simulink model "evse_twin_shit"  (R2023b)
settings: Solver=VariableStepAuto  StartTime=0.0  StopTime=5  RelTol=1e-3
libraries: fl_lib x14, nesl_utility x7
settings Model: Creator=dawid  LastModifiedBy=dawid
settings OptimizationCC: BooleanDataType=off

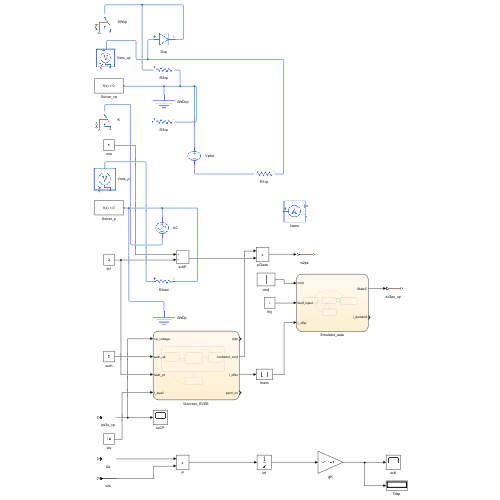
[thumbnail: Simulink's stored preview of the top-level diagram]
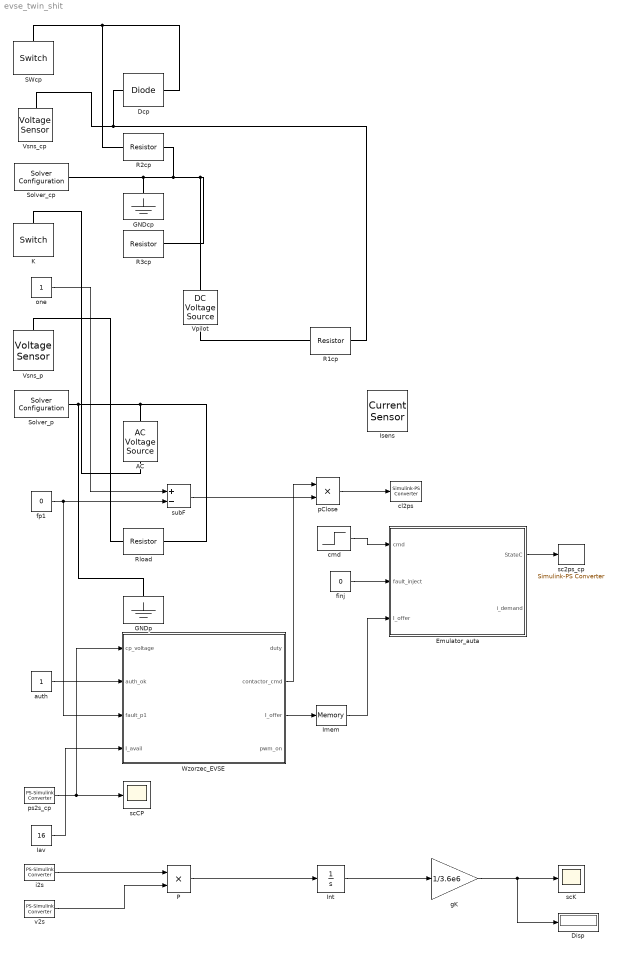
== system evse_twin_shit ==
  AC : fl_lib/Electrical/Electrical Sources/AC Voltage Source  amp=1 V  shift=0 deg  frequency=50 Hz  omega=0 rad/s
  Dcp : fl_lib/Electrical/Electrical Elements/Diode  Vf=0.6 V  Ron=0.3 Ohm  Goff=1e-8 1/Ohm  i_specify=off  i_priority=None  i=0 A  i_nominal_specify=off  i_nominal_unit=A  i_nominal_value=1  v_specify=off  v_priority=None  v=0 V  v_nominal_specify=off  v_nominal_unit=V  v_nominal_value=1
  Disp : Display
  Emulator_auta : Stateflow chart  TreatAsAtomicUnit=on
  GNDcp : fl_lib/Electrical/Electrical Elements/Electrical Reference
  GNDp : fl_lib/Electrical/Electrical Elements/Electrical Reference
  Iav : Constant  Value=16
  Imem : Memory
  Int : Integrator
  Isens : fl_lib/Electrical/Electrical Sensors/Current Sensor
  K : fl_lib/Electrical/Electrical Elements/Switch  R_closed=0.01 Ohm  G_open=1e-8 1/Ohm  Threshold=0.5  i_specify=off  i_priority=None  i=0 A  i_nominal_specify=off  i_nominal_unit=A  i_nominal_value=1  v_specify=off  v_priority=None  v=0 V  v_nominal_specify=off  v_nominal_unit=V  v_nominal_value=1
  P : Product
  R1cp : fl_lib/Electrical/Electrical Elements/Resistor  R=1000 Ohm  i_specify=off  i_priority=None  i=0 A  i_nominal_specify=off  i_nominal_unit=A  i_nominal_value=1  v_specify=off  v_priority=None  v=0 V  v_nominal_specify=off  v_nominal_unit=V  v_nominal_value=1
  R2cp : fl_lib/Electrical/Electrical Elements/Resistor  R=2740 Ohm  i_specify=off  i_priority=None  i=0 A  i_nominal_specify=off  i_nominal_unit=A  i_nominal_value=1  v_specify=off  v_priority=None  v=0 V  v_nominal_specify=off  v_nominal_unit=V  v_nominal_value=1
  R3cp : fl_lib/Electrical/Electrical Elements/Resistor  R=1300 Ohm  i_specify=off  i_priority=None  i=0 A  i_nominal_specify=off  i_nominal_unit=A  i_nominal_value=1  v_specify=off  v_priority=None  v=0 V  v_nominal_specify=off  v_nominal_unit=V  v_nominal_value=1
  Rload : fl_lib/Electrical/Electrical Elements/Resistor  R=14.4 Ohm  i_specify=off  i_priority=None  i=0 A  i_nominal_specify=off  i_nominal_unit=A  i_nominal_value=1  v_specify=off  v_priority=None  v=0 V  v_nominal_specify=off  v_nominal_unit=V  v_nominal_value=1
  SWcp : fl_lib/Electrical/Electrical Elements/Switch  R_closed=0.01 Ohm  G_open=1e-8 1/Ohm  Threshold=0.5  i_specify=off  i_priority=None  i=0 A  i_nominal_specify=off  i_nominal_unit=A  i_nominal_value=1  v_specify=off  v_priority=None  v=0 V  v_nominal_specify=off  v_nominal_unit=V  v_nominal_value=1
  Solver_cp : nesl_utility/Solver Configuration  PhysicalDomain=network_engine_domain  SubClassName=solver  LeftPortType=input  RightPortType=generic  Tones=[]  Harmonics=[]  SimulateNoise=off  Profile=off  UseLocalSampling=off  EnableSwitchedLinearOptims=on  FrequencyDomain=off  UseCCode=off  RelTol=0.001  AbsTol=0.001  MinStep=1e-09  ToWorkspace=off  RevertToSquareIcSolve=off  NumHomotopyIterations=100  PhasorMode=off  PhasorModeNumHarmonics=1  ConsistencySolver=NEWTON_XTOL_AFTER_FTOL  IndexReductionMethod=DerivativeReplacement  DoDC=off  ResidualTolerance=1e-09  ConsistencyTolSource=GLOBAL  ConsistencyAbsTol=0.001  ConsistencyRelTol=0.001  ConsistencyTolFactor=0.001  UseLocalSolver=off  LocalSolverChoice=NE_BACKWARD_EULER_ADVANCER  ResolveIndetEquations=on  FunctionEvalNumThread=1  LocalSolverSampleTime=0.001  DoFixedCost=off  MaxNonlinIter=3  MaxModeIter=2  ComputeImpulses=off  ImpulseIterations=2  LinearAlgebra=auto  LinearAlgebraNumThread=0  EquationFormulation=NE_TIME_EF  DelaysMemoryBudget=1024  AutomaticFiltering=on  FilteringTimeConstant=0.001  PartitionStorageMethod=AS_NEEDED  PartitionMemoryBudget=1024  PartitionMethod=ROBUST  MultibodyUseLocalSolver=off  MultibodyLocalSolverChoice=ODE1  MultibodyLocalSolverSampleTime=0.001
  Solver_p : nesl_utility/Solver Configuration  PhysicalDomain=network_engine_domain  SubClassName=solver  LeftPortType=input  RightPortType=generic  Tones=[]  Harmonics=[]  SimulateNoise=off  Profile=off  UseLocalSampling=off  EnableSwitchedLinearOptims=on  FrequencyDomain=off  UseCCode=off  RelTol=0.001  AbsTol=0.001  MinStep=1e-09  ToWorkspace=off  RevertToSquareIcSolve=off  NumHomotopyIterations=100  PhasorMode=off  PhasorModeNumHarmonics=1  ConsistencySolver=NEWTON_XTOL_AFTER_FTOL  IndexReductionMethod=DerivativeReplacement  DoDC=off  ResidualTolerance=1e-09  ConsistencyTolSource=GLOBAL  ConsistencyAbsTol=0.001  ConsistencyRelTol=0.001  ConsistencyTolFactor=0.001  UseLocalSolver=off  LocalSolverChoice=NE_BACKWARD_EULER_ADVANCER  ResolveIndetEquations=on  FunctionEvalNumThread=1  LocalSolverSampleTime=0.001  DoFixedCost=off  MaxNonlinIter=3  MaxModeIter=2  ComputeImpulses=off  ImpulseIterations=2  LinearAlgebra=auto  LinearAlgebraNumThread=0  EquationFormulation=NE_TIME_EF  DelaysMemoryBudget=1024  AutomaticFiltering=on  FilteringTimeConstant=0.001  PartitionStorageMethod=AS_NEEDED  PartitionMemoryBudget=1024  PartitionMethod=ROBUST  MultibodyUseLocalSolver=off  MultibodyLocalSolverChoice=ODE1  MultibodyLocalSolverSampleTime=0.001
  Vpilot : fl_lib/Electrical/Electrical Sources/DC Voltage Source  v0=12 V
  Vsns_cp : fl_lib/Electrical/Electrical Sensors/Voltage Sensor
  Vsns_p : fl_lib/Electrical/Electrical Sensors/Voltage Sensor
  Wzorzec_EVSE : Stateflow chart  TreatAsAtomicUnit=on
  auth : Constant
  cl2ps : nesl_utility/Simulink-PS Converter  PhysicalDomain=network_engine_domain  SubClassName=ps_input  LeftPortType=input  RightPortType=output  PseudoPeriodic=off  Frequencies=[]  NoiseDistribution=none  NoiseParameters=[]  Unit=1  AffineConversion=off  FilteringAndDerivatives=provide  SimscapeFilterOrder=1  InputFilterTimeConstant=0.001  UdotUserProvided=0
  cmd : Step  Time=2  Before=1  After=2  SampleTime=0
  finj : Constant  Value=0
  fp1 : Constant  Value=0
  gK : Gain  Gain=1/3.6e6
  i2s : nesl_utility/PS-Simulink Converter  PhysicalDomain=network_engine_domain  SubClassName=ps_output  LeftPortType=input  RightPortType=output  PseudoPeriodic=off  Frequencies=[]  VectorFormat=inherit  Unit=inherit  AffineConversion=off
  one : Constant
  pClose : Product
  ps2s_cp : nesl_utility/PS-Simulink Converter  PhysicalDomain=network_engine_domain  SubClassName=ps_output  LeftPortType=input  RightPortType=output  PseudoPeriodic=off  Frequencies=[]  VectorFormat=inherit  Unit=inherit  AffineConversion=off
  sc2ps_cp : nesl_utility/Simulink-PS Converter  PhysicalDomain=network_engine_domain  SubClassName=ps_input  LeftPortType=input  RightPortType=output  PseudoPeriodic=off  Frequencies=[]  NoiseDistribution=none  NoiseParameters=[]  Unit=1  AffineConversion=off  FilteringAndDerivatives=provide  SimscapeFilterOrder=1  InputFilterTimeConstant=0.001  UdotUserProvided=0
  scCP : Scope
  scK : Scope
  subF : Sum  Inputs=+-
  v2s : nesl_utility/PS-Simulink Converter  PhysicalDomain=network_engine_domain  SubClassName=ps_output  LeftPortType=input  RightPortType=output  PseudoPeriodic=off  Frequencies=[]  VectorFormat=inherit  Unit=inherit  AffineConversion=off
  wires:
  one/1 -> subF/1
  fp1/1 -> Wzorzec_EVSE/3(fault_p1), subF/2
  auth/1 -> Wzorzec_EVSE/2(auth_ok)
  ps2s_cp/1 -> Wzorzec_EVSE/1(cp_voltage), scCP/1
  Iav/1 -> Wzorzec_EVSE/4(I_avail)
  i2s/1 -> P/1
  Imem/1 -> Emulator_auta/3(I_offer)
  v2s/1 -> P/2
  P/1 -> Int/1
  subF/1 -> pClose/2
  Wzorzec_EVSE/2(contactor_cmd) -> pClose/1
  Wzorzec_EVSE/3(I_offer) -> Imem/1
  pClose/1 -> cl2ps/1
  cmd/1 -> Emulator_auta/1(cmd)
  finj/1 -> Emulator_auta/2(fault_inject)
  Int/1 -> gK/1
  Emulator_auta/1(StateC) -> sc2ps_cp/1
  gK/1 -> Disp/1, scK/1
  connections:
  Vpilot/RConn1 -- R1cp/LConn1
  Solver_cp/RConn1 -- R3cp/RConn1 -- Vpilot/LConn1 -- R2cp/RConn1 -- GNDcp/LConn1
  Vsns_cp/LConn1 -- R1cp/RConn1 -- Dcp/LConn1
  SWcp/LConn1 -- R2cp/LConn1 -- Dcp/RConn1
  K/LConn1 -- AC/RConn1
  Solver_p/RConn1 -- AC/LConn1 -- Rload/RConn1 -- GNDp/LConn1
  Vsns_p/LConn1 -- Rload/LConn1

== stateflow chart evse_twin_shit/Wzorzec_EVSE ==
  state Operating
    state Idle
      entry: pwm_on=0; duty=0; contactor_cmd=0; I_offer=0;
    state Detected
      entry: pwm_on=1; I_offer=I_avail; duty=max(10,min(85,I_offer/0.6)); contactor_cmd=0;
    state Charging
      entry: contactor_cmd=1;
      during: I_offer=I_avail; duty=max(10,min(85,I_offer/0.6));
    Charging -> Detected : [cp_voltage>7.5 && cp_voltage<10.5]
    (default) -> Idle
    Detected -> Charging [order 1] : [cp_voltage>4.5 && cp_voltage<7.5 && auth_ok==1]
    Idle -> Detected : [cp_voltage>7.5 && cp_voltage<10.5 && I_avail>0]
    Detected -> Idle [order 2] : [cp_voltage>10.5]
  state Tripped
    entry: contactor_cmd=0; pwm_on=0; duty=0;
  Tripped -> Operating : [fault_p1==0 && cp_voltage>1.5]
  Operating -> Tripped : [fault_p1==1 || cp_voltage<1.5]
  data: cp_voltage input; auth_ok input; fault_p1 input; I_avail input; duty output; contactor_cmd output; I_offer output; pwm_on output

== stateflow chart evse_twin_shit/Emulator_auta ==
  state A_Unplugged
    entry: StateC=0; i_demand=0;
  state B_Connected
    entry: StateC=0; i_demand=0;
  state C_Ready
    entry: StateC=1; i_demand=min(I_offer,32);
  state Fault
    entry: StateC=0; i_demand=0;
  C_Ready -> A_Unplugged [order 2] : [cmd==0]
  (default) -> A_Unplugged
  C_Ready -> B_Connected [order 1] : [cmd==3]
  C_Ready -> Fault [order 3] : [fault_inject==1]
  A_Unplugged -> B_Connected : [cmd==1]
  B_Connected -> C_Ready [order 1] : [cmd==2]
  B_Connected -> A_Unplugged [order 2] : [cmd==0]
  Fault -> A_Unplugged : [fault_inject==0]
  B_Connected -> Fault [order 3] : [fault_inject==1]
  data: cmd input; fault_inject input; I_offer input; StateC output; i_demand output
